simulink model "testConvPACKET"  (R2024b)
settings: Solver=VariableStepAuto  StartTime=0.0  StopTime=10.0  RelTol=1e-3
undefined symbols (not defined in the file or in its folder): Param
libraries: simulink x2, commcnvcod2 x1, commblkintrlv2 x1
settings Model: Creator=SERGIO  LastModifiedBy=SERGIO

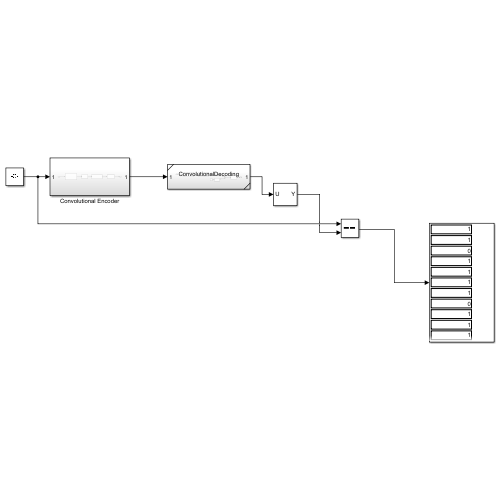
[thumbnail: Simulink's stored preview of the top-level diagram]
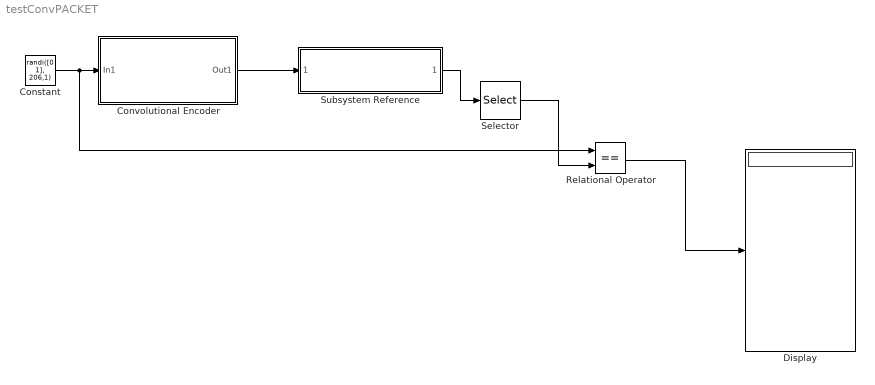
== system testConvPACKET ==
  Constant : Constant  Value=randi([0 1], 206,1)  VectorParams1D=off
  Convolutional Encoder : Subsystem
  Display : Display
  Relational Operator : RelationalOperator  Operator===  OutDataTypeStr=boolean  RndMeth=Simplest  InputSameDT=off
  Selector : Selector  IndexOptions=Index vector (dialog)  Indices=[1:206]  OutputSizes=1
  Subsystem Reference : Subsystem  ReferencedSubsystem=ConvolutionalDecoding
  wires:
  Convolutional Encoder/1(Out1) -> Subsystem Reference/1
  Constant/1 -> Relational Operator/1, Convolutional Encoder/1(In1)
  Relational Operator/1 -> Display/1
  Subsystem Reference/1 -> Selector/1
  Selector/1 -> Relational Operator/2

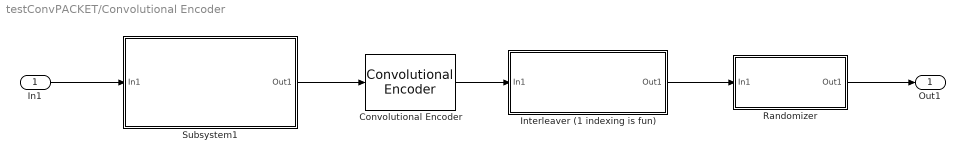
== system testConvPACKET/Convolutional Encoder ==
  In1 : Inport
  Convolutional Encoder : commcnvcod2/Convolutional Encoder  trellis=poly2trellis(5, [23 35])  opMode=Truncated (reset every frame)  DelayedResetAction=on  hasIniStPort=off  hasFinStPort=off  usePuncVector=on  punctureVector=Param.Puncturing.P3  reset=Unused parameter value
  Interleaver (1 indexing is fun) : Subsystem
  Randomizer : Subsystem
  Subsystem1 : Subsystem
  Out1 : Outport
  wires:
  Randomizer/1(Out1) -> Out1/1
  Convolutional Encoder/1 -> Interleaver (1 indexing is fun)/1(In1)
  Interleaver (1 indexing is fun)/1(Out1) -> Randomizer/1(In1)
  Subsystem1/1(Out1) -> Convolutional Encoder/1
  In1/1 -> Subsystem1/1(In1)

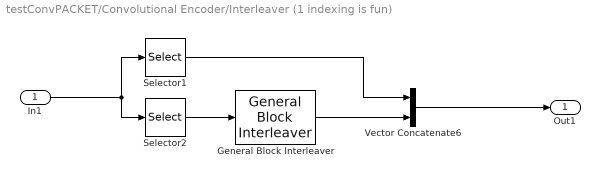
== system testConvPACKET/Convolutional Encoder/Interleaver (1 indexing is fun) ==
  In1 : Inport
  General Block Interleaver : commblkintrlv2/General Block Interleaver  StatePerturbationForJacobian=1.0e-05  permutationVectorSource=Dialog  elements=Param.InterleavingTable
  Selector1 : Selector  IndexOptions=Index vector (dialog)  Indices=[1]  OutputSizes=1
  Selector2 : Selector  IndexOptions=Index vector (dialog)  Indices=[2:368]  OutputSizes=1
  Vector Concatenate6 : Concatenate
  Out1 : Outport
  wires:
  Vector Concatenate6/1 -> Out1/1
  Selector2/1 -> General Block Interleaver/1
  In1/1 -> Selector1/1, Selector2/1
  Selector1/1 -> Vector Concatenate6/1
  General Block Interleaver/1 -> Vector Concatenate6/2

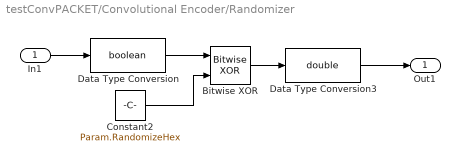
== system testConvPACKET/Convolutional Encoder/Randomizer ==
  In1 : Inport
  Bitwise XOR : simulink/Logic and Bit Operations/Bitwise Operator  logicop=XOR  UseBitMask=off  NumInputPorts=2  BitMask=bin2dec('11011001')  BitMaskRealWorld=Stored Integer
  Constant2 : Constant  Value=Param.RandomizeHex  VectorParams1D=off
  Data Type Conversion : DataTypeConversion  OutDataTypeStr=boolean  SaturateOnIntegerOverflow=off  RndMeth=Floor
  Data Type Conversion3 : DataTypeConversion  OutDataTypeStr=double  SaturateOnIntegerOverflow=off  RndMeth=Floor
  Out1 : Outport
  wires:
  Bitwise XOR/1 -> Data Type Conversion3/1
  Constant2/1 -> Bitwise XOR/2
  In1/1 -> Data Type Conversion/1
  Data Type Conversion3/1 -> Out1/1
  Data Type Conversion/1 -> Bitwise XOR/1

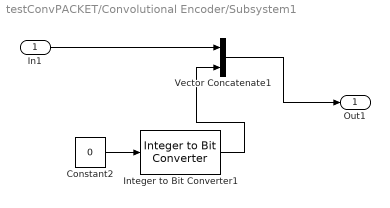
== system testConvPACKET/Convolutional Encoder/Subsystem1 ==
  In1 : Inport
  Constant2 : Constant  Value=0
  Integer to Bit Converter1 : simulink/Logic and Bit Operations/Integer to Bit Converter  nbits=6  signedInputValues=Unsigned  bitOrder=MSB first  outDtype=Inherit via internal rule
  Vector Concatenate1 : Concatenate
  Out1 : Outport
  wires:
  In1/1 -> Vector Concatenate1/1
  Integer to Bit Converter1/1 -> Vector Concatenate1/2
  Constant2/1 -> Integer to Bit Converter1/1
  Vector Concatenate1/1 -> Out1/1
